simulink model "Lab07"  (R2024b)
settings: Solver=VariableStepAuto  StartTime=0.0  StopTime=10.0  RelTol=1e-3
values from neighbouring files (symbols this model uses):
  I = diag(Iv)    [initLab7.m]
  invI = inv(I)    [initLab7.m]
  w0 = [0; 0; 0]    [initLab7.m]
undefined symbols (not defined in the file or in its folder): env, IC, orb, sat, WMM2020
libraries: matrix_library x8, aerolibatmos2 x1, aerolibgravity2 x1
settings Model: Creator=elisa  LastModifiedBy=elisa
settings RTWCC: GPUComputeCapability=3.5

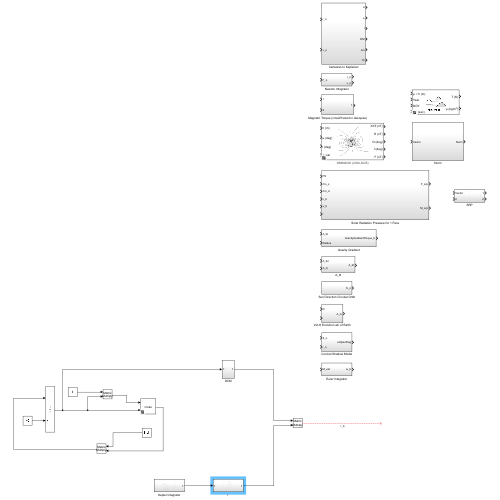
[thumbnail: Simulink's stored preview of the top-level diagram]
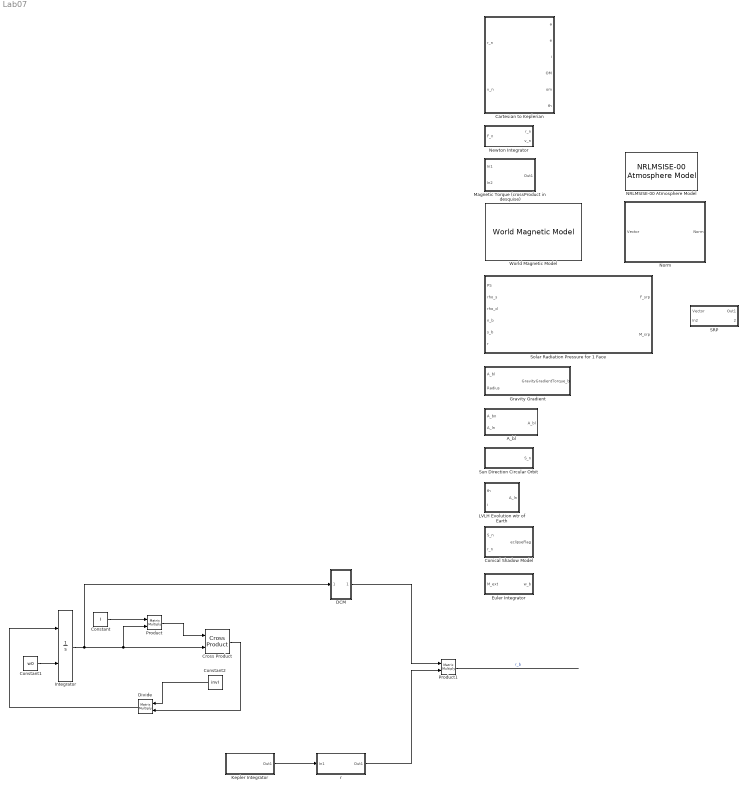
== system Lab07 ==
  A_bl : Subsystem
  Cartesian to Keplerian : Subsystem
  Conical Shadow Model : Subsystem
  Constant : Constant  Value=I
  Constant1 : Constant  Value=w0  VectorParams1D=off
  Constant2 : Constant  Value=invI
  Cross Product : matrix_library/Cross Product
  DCM : Subsystem
  Divide : Product  Inputs=**  Multiplication=Matrix(*)
  Euler Integrator : Subsystem
  Gravity Gradient : Subsystem
  Integrator : Integrator  InitialConditionSource=external
  Kepler Integrator : Subsystem
  LVLH Evolution wtr of Earth : Subsystem
  Magnetic Torque (crossProduct in desquise) : Subsystem
  NRLMSISE-00 Atmosphere Model : aerolibatmos2/NRLMSISE-00 Atmosphere Model  units=Metric (MKS)  lst_input=off  flux_ap_input=off  flags_input=Internal  flags=ones(1,23)  oxygen_in=off  action=Warning
  Newton Integrator : Subsystem
  Norm : Subsystem
  Product : Product  Multiplication=Matrix(*)
  Product1 : Product  Multiplication=Matrix(*)
  SRP : Subsystem
  Solar Radiation Pressure for 1 Face : Subsystem
  Sun Direction Circular Orbit : Subsystem
  World Magnetic Model : aerolibgravity2/World Magnetic Model  model=WMM2020 (2020-2025)  customFile='WMM2020.COF'  units=Metric (MKS)  time_in=on  month=January  day=1  year=2020  action=Error  h_out=on  dec_out=on  inc_out=on  ti_out=on
  r : Subsystem
  wires:
  Kepler Integrator/1(Out1) -> r/1(In1)
  Divide/1 -> Integrator/1
  Constant2/1 -> Divide/1
  Integrator/1 -> DCM/1(In1), Product/2, Cross Product/2
  Product/1 -> Cross Product/1
  Cross Product/1 -> Divide/2
  Constant1/1 -> Integrator/2
  Constant/1 -> Product/1
  DCM/1(Out1) -> Product1/1
  r/1(Out1) -> Product1/2
  Product1/1 -> ?  "r_b"

== system Lab07/A_bl ==
  A_bn : Inport
  A_ln : Inport  Port=2
  Matrix Multiply : Product  Multiplication=Matrix(*)
  Transpose : Math  Operator=transpose
  A_bl : Outport
  wires:
  Transpose/1 -> Matrix Multiply/2
  A_ln/1 -> Transpose/1
  Matrix Multiply/1 -> A_bl/1
  A_bn/1 -> Matrix Multiply/1

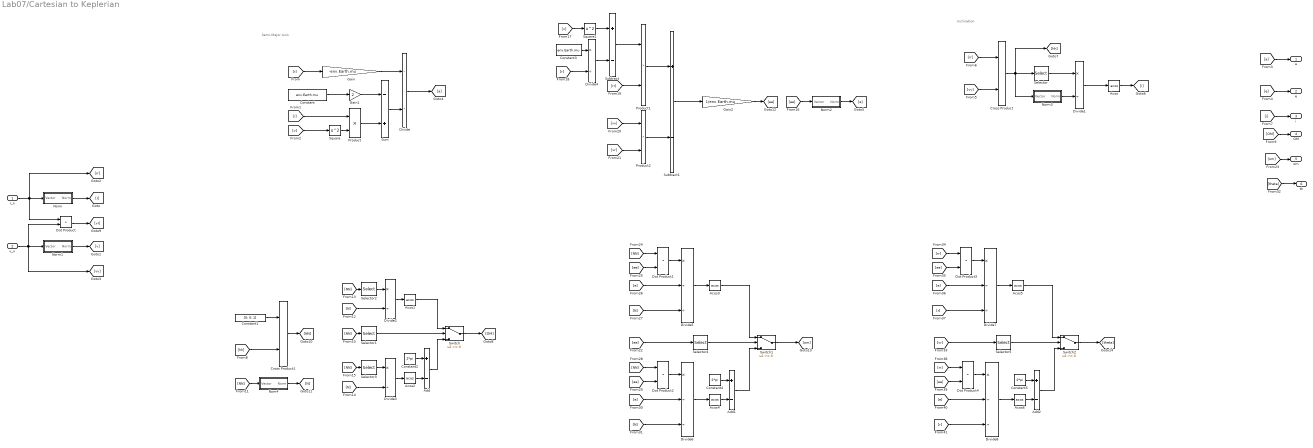
== system Lab07/Cartesian to Keplerian ==
  note: Semi-Major Axis
  note: Inclination
  r_n : Inport
  v_n : Inport  Port=2
  Acos{,1..6} (7 alike) : Trigonometry  Operator=acos
  Add : Sum  Inputs=+-
  Add1 : Sum  Inputs=+-
  Add2 : Sum  Inputs=+-
  Constant : Constant  Value=env.Earth.mu
  Constant1 : Constant  Value=[0; 0; 1]
  Constant2 : Constant  Value=2*pi
  Constant3 : Constant  Value=env.Earth.mu
  Constant4 : Constant  Value=2*pi
  Constant5 : Constant  Value=2*pi
  Cross Product : matrix_library/Cross Product
  Cross Product1 : matrix_library/Cross Product
  Divide{,1..4} (5 alike) : Product  Inputs=*/
  Divide{5..8} (4 alike) : Product  Inputs=*//
  Dot Product{,1..4} (5 alike) : DotProduct  OutDataTypeStr=Inherit: Inherit via internal rule
  Gain : Gain  Gain=-env.Earth.mu
  Gain1 : Gain  Gain=2
  Gain2 : Gain  Gain=1/env.Earth.mu
  Nom4 : Subsystem
  Norm : Subsystem
  Norm1 : Subsystem
  Norm2 : Subsystem
  Norm3 : Subsystem
  Product : Product
  Product1 : Product
  Product2 : Product
  Selector : Selector  InputPortWidth=3  IndexOptions=Index vector (dialog)  Indices=[3]  OutputSizes=1
  Selector1 : Selector  InputPortWidth=3  IndexOptions=Index vector (dialog)  Indices=[2]  OutputSizes=1
  Selector2 : Selector  InputPortWidth=3  IndexOptions=Index vector (dialog)  Indices=[1]  OutputSizes=1
  Selector3 : Selector  InputPortWidth=3  IndexOptions=Index vector (dialog)  Indices=[1]  OutputSizes=1
  Selector4 : Selector  InputPortWidth=3  IndexOptions=Index vector (dialog)  Indices=3  OutputSizes=1
  Selector5 : Selector  InputPortWidth=3  IndexOptions=Index vector (dialog)  Indices=3  OutputSizes=1
  Square : Math  Operator=square
  Square1 : Math  Operator=square
  Subtract : Sum  Inputs=+-
  Subtract1 : Sum  Inputs=+-
  Sum : Sum  Inputs=-+
  Switch : Switch  SaturateOnIntegerOverflow=off  InputSameDT=off
  Switch1 : Switch  SaturateOnIntegerOverflow=off  InputSameDT=off
  Switch2 : Switch  SaturateOnIntegerOverflow=off  InputSameDT=off
  a : Outport
  e : Outport  Port=2
  i : Outport  Port=3
  OM : Outport  Port=4
  om : Outport  Port=5
  th : Outport  Port=6
  wires:
  r_n/1 -> Dot Product/1, [rr], Norm/1(Vector)
  v_n/1 -> Dot Product/2, [vv], Norm1/1(Vector)
  Norm/1(Norm) -> [r]
  Norm1/1(Norm) -> [v]
  Gain/1 -> Divide/1
  [r] -> Gain/1
  Sum/1 -> Divide/2
  Constant/1 -> Gain1/1
  Gain1/1 -> Sum/1
  Product/1 -> Sum/2
  [r] -> Product/1
  Square/1 -> Product/2
  [v] -> Square/1
  Divide/1 -> [a]
  [a] -> a/1
  Norm2/1(Norm) -> [e]
  [e] -> e/1
  [vv] -> Cross Product/2
  [rr] -> Cross Product/1
  Cross Product/1 -> [hh], Norm3/1(Vector), Selector/1
  Selector/1 -> Divide1/1
  Norm3/1(Norm) -> Divide1/2
  Divide1/1 -> Acos/1
  Acos/1 -> [i]
  [i] -> i/1
  [hh] -> Cross Product1/2
  Constant1/1 -> Cross Product1/1
  Selector1/1 -> Switch/2
  [OM] -> OM/1
  Switch/1 -> [OM]
  Dot Product/1 -> [vr]
  Cross Product1/1 -> [NN]
  [NN] -> Selector1/1
  [NN] -> Nom4/1(Vector)
  Nom4/1(Norm) -> [N]
  [NN] -> Selector2/1
  [N] -> Divide2/2
  Selector2/1 -> Divide2/1
  Acos1/1 -> Switch/1
  Selector3/1 -> Divide3/1
  [NN] -> Selector3/1
  [N] -> Divide3/2
  Divide3/1 -> Acos2/1
  Divide2/1 -> Acos1/1
  Acos2/1 -> Add/2
  Constant2/1 -> Add/1
  Add/1 -> Switch/3
  [ee] -> Norm2/1(Vector)
  Gain2/1 -> [ee]
  [v] -> Square1/1
  Constant3/1 -> Divide4/1
  [r] -> Divide4/2
  Divide4/1 -> Subtract/2
  Square1/1 -> Subtract/1
  Subtract/1 -> Product1/1
  [rr] -> Product1/2
  Product1/1 -> Subtract1/1
  Product2/1 -> Subtract1/2
  [vv] -> Product2/1
  [vr] -> Product2/2
  Subtract1/1 -> Gain2/1
  Selector4/1 -> Switch1/2
  [ee] -> Selector4/1
  Switch1/1 -> [om]
  [om] -> om/1
  [NN] -> Dot Product1/1
  [ee] -> Dot Product1/2
  Dot Product1/1 -> Divide5/1
  [e] -> Divide5/2
  [N] -> Divide5/3
  Divide5/1 -> Acos3/1
  Acos3/1 -> Switch1/1
  [ee] -> Dot Product2/2
  Divide6/1 -> Acos4/1
  Dot Product2/1 -> Divide6/1
  [NN] -> Dot Product2/1
  [N] -> Divide6/3
  [e] -> Divide6/2
  Constant4/1 -> Add1/1
  Acos4/1 -> Add1/2
  Add1/1 -> Switch1/3
  [vr] -> Selector5/1
  Switch2/1 -> [theta]
  Selector5/1 -> Switch2/2
  [theta] -> th/1
  [ee] -> Dot Product3/2
  Divide7/1 -> Acos5/1
  Dot Product3/1 -> Divide7/1
  [rr] -> Dot Product3/1
  [r] -> Divide7/3
  Acos5/1 -> Switch2/1
  [e] -> Divide7/2
  Add2/1 -> Switch2/3
  [rr] -> Dot Product4/1
  [r] -> Divide8/3
  Dot Product4/1 -> Divide8/1
  [e] -> Divide8/2
  Acos6/1 -> Add2/2
  Constant5/1 -> Add2/1
  Divide8/1 -> Acos6/1
  [ee] -> Dot Product4/2

== system Lab07/Conical Shadow Model ==
  note: Output Interface
  note: Input Interface
  note: Model is cylindrical shadow, formula was taken by Crassidis
  S_n : Inport
  r_n : Inport  Port=2
  Dot Product : DotProduct  OutDataTypeStr=Inherit: Inherit via internal rule
  Earth's Radius : Constant  Value=env.Earth.R
  Eclipse (1) : Subsystem  TreatAsAtomicUnit=on
  Gain : Gain  Gain=-1
  If : If  NumInputs=2  IfExpression=u1 < u2
  Merge : Merge
  Norm : Subsystem
  NotEclipse (0) : Subsystem  TreatAsAtomicUnit=on
  Sqrt : Sqrt
  Square : Math  Operator=square
  Square1 : Math  Operator=square
  Subtract : Sum  Inputs=+-
  eclipseFlag : Outport
  wires:
  r_n/1 -> Dot Product/2, Norm/1(Vector)  "r_n"
  S_n/1 -> Dot Product/1  "S_n"
  Norm/1(Norm) -> Square1/1  "norm_r"
  If/1 -> Eclipse (1)/Action
  If/2 -> NotEclipse (0)/Action
  Merge/1 -> eclipseFlag/1
  Eclipse (1)/1(One) -> Merge/1
  NotEclipse (0)/1(Zero) -> Merge/2
  Dot Product/1 -> If/1
  Gain/1 -> If/2
  Sqrt/1 -> Gain/1
  Subtract/1 -> Sqrt/1
  Square/1 -> Subtract/2
  Square1/1 -> Subtract/1
  Earth's Radius/1 -> Square/1  "earth_R"

== system Lab07/DCM ==
  In1 : Inport
  A312 : Subsystem
  Constant3 : Constant  Value=IC.angles
  Gain : Gain  Gain=-1
  Integrator1 : Integrator  InitialConditionSource=external
  Product1 : Product  Multiplication=Matrix(*)
  Subsystem : Subsystem
  Subsystem1 : Subsystem
  Subsystem2 : Subsystem
  w^ : Subsystem
  Out1 : Outport
  wires:
  w^/1(Out1) -> Gain/1
  Gain/1 -> Product1/1
  In1/1 -> w^/1(In1)
  Product1/1 -> Integrator1/1
  Constant3/1 -> A312/1(In1)
  Integrator1/1 -> Subsystem/1(In1)
  Subsystem/1(Out1) -> Subsystem1/1(In1)
  A312/1(Out1) -> Integrator1/2
  Subsystem1/1(Out1) -> Subsystem2/1(In1)
  Subsystem2/1(Out1) -> Product1/2, Out1/1

== system Lab07/Euler Integrator ==
  M_ext : Inport
  Constant : Constant  Value=I
  Constant1 : Constant  Value=w0  VectorParams1D=off
  Constant2 : Constant  Value=invI
  Cross Product : matrix_library/Cross Product
  Divide : Product  Inputs=**  Multiplication=Matrix(*)
  Integrator : Integrator  InitialConditionSource=external
  Product : Product  Multiplication=Matrix(*)
  Sum : Sum  Inputs=|++
  w_b : Outport
  wires:
  Product/1 -> Cross Product/1
  Divide/1 -> Integrator/1
  Constant/1 -> Product/1
  Constant2/1 -> Divide/1
  Integrator/1 -> Product/2, Cross Product/2, w_b/1
  Constant1/1 -> Integrator/2
  Cross Product/1 -> Sum/1
  Sum/1 -> Divide/2
  M_ext/1 -> Sum/2

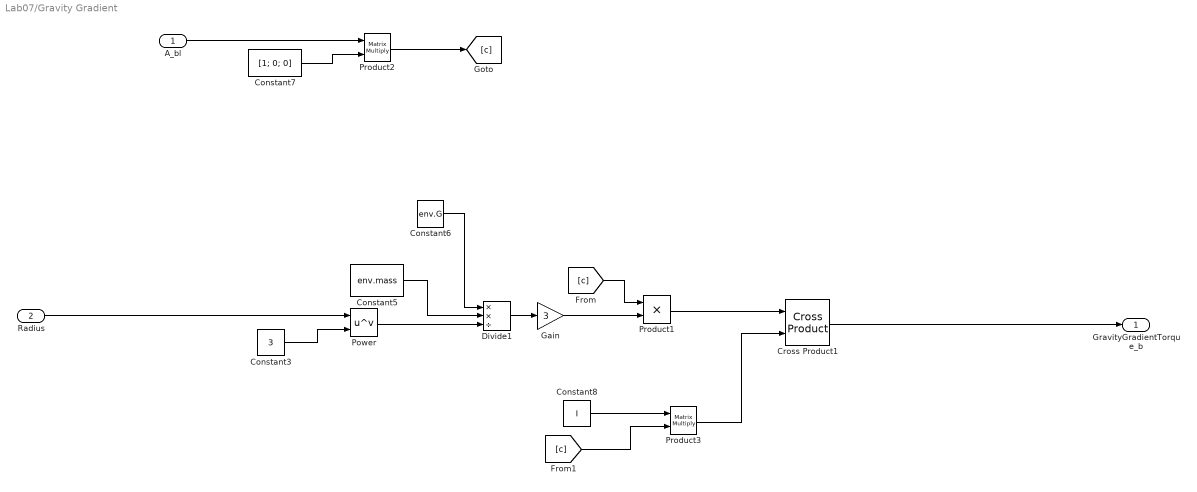
== system Lab07/Gravity Gradient ==
  A_bl : Inport
  Radius : Inport  Port=2
  Constant3 : Constant  Value=3
  Constant5 : Constant  Value=env.mass
  Constant6 : Constant  Value=env.G
  Constant7 : Constant  Value=[1; 0; 0]  VectorParams1D=off
  Constant8 : Constant  Value=I
  Cross Product1 : matrix_library/Cross Product
  Divide1 : Product  Inputs=**/
  Gain : Gain  Gain=3
  Power : Math  Operator=pow
  Product1 : Product
  Product2 : Product  Multiplication=Matrix(*)
  Product3 : Product  Multiplication=Matrix(*)
  GravityGradientTorque_b : Outport
  wires:
  Divide1/1 -> Gain/1
  Power/1 -> Divide1/3
  Constant3/1 -> Power/2
  Constant7/1 -> Product2/2
  Radius/1 -> Power/1
  Constant5/1 -> Divide1/2
  Constant6/1 -> Divide1/1
  [c] -> Product3/2
  [c] -> Product1/1
  Product1/1 -> Cross Product1/1
  Cross Product1/1 -> GravityGradientTorque_b/1
  Constant8/1 -> Product3/1
  Product2/1 -> [c]
  Product3/1 -> Cross Product1/2
  A_bl/1 -> Product2/1
  Gain/1 -> Product1/2

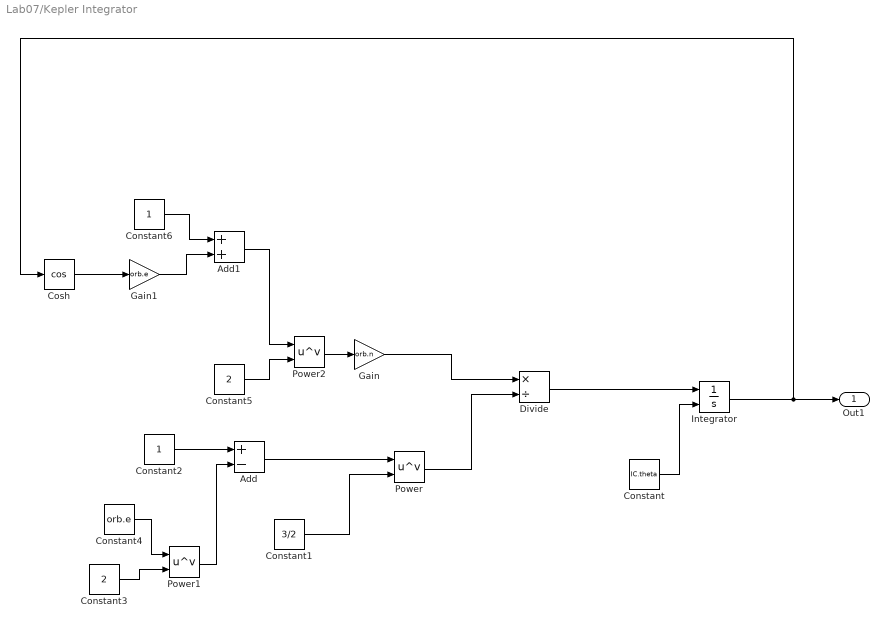
== system Lab07/Kepler Integrator ==
  Add : Sum  Inputs=+-
  Add1 : Sum
  Constant : Constant  Value=IC.theta
  Constant1 : Constant  Value=3/2
  Constant2 : Constant
  Constant3 : Constant  Value=2
  Constant4 : Constant  Value=orb.e
  Constant5 : Constant  Value=2
  Constant6 : Constant
  Cosh : Trigonometry  Operator=cos
  Divide : Product  Inputs=*/
  Gain : Gain  Gain=orb.n
  Gain1 : Gain  Gain=orb.e
  Integrator : Integrator  InitialConditionSource=external  WrapState=on  WrappedStateUpperValue=2*pi  WrappedStateLowerValue=0
  Power : Math  Operator=pow
  Power1 : Math  Operator=pow
  Power2 : Math  Operator=pow
  Out1 : Outport
  wires:
  Constant/1 -> Integrator/2
  Integrator/1 -> Cosh/1, Out1/1
  Divide/1 -> Integrator/1
  Power/1 -> Divide/2
  Constant1/1 -> Power/2
  Constant2/1 -> Add/1
  Add/1 -> Power/1
  Power1/1 -> Add/2
  Constant3/1 -> Power1/2
  Constant4/1 -> Power1/1
  Gain/1 -> Divide/1
  Power2/1 -> Gain/1
  Constant5/1 -> Power2/2
  Add1/1 -> Power2/1
  Constant6/1 -> Add1/1
  Gain1/1 -> Add1/2
  Cosh/1 -> Gain1/1

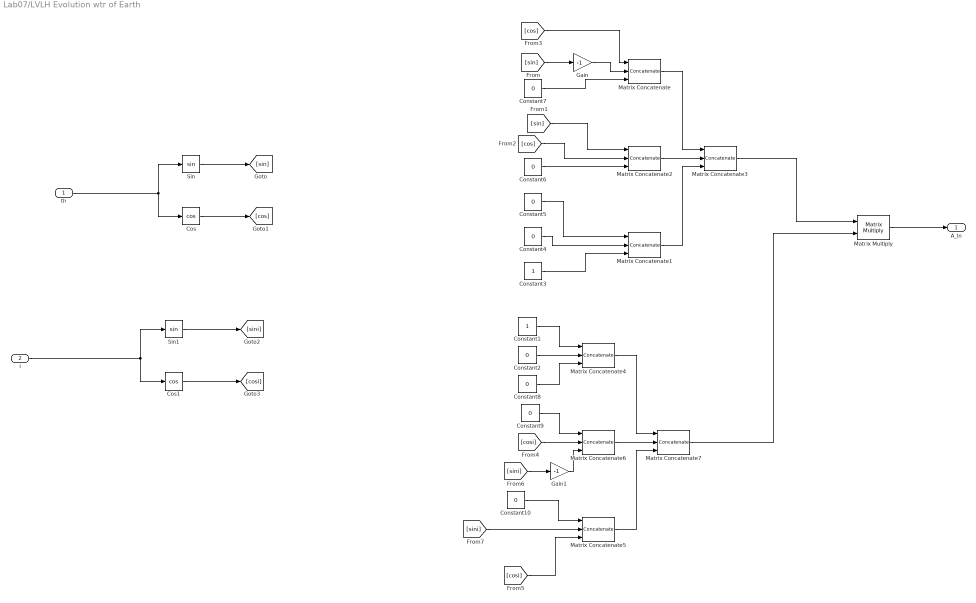
== system Lab07/LVLH Evolution wtr of Earth ==
  th : Inport
  i : Inport  Port=2
  Constant1 : Constant
  Constant{2,4..10} (8 alike) : Constant  Value=0
  Constant3 : Constant
  Cos : Trigonometry  Operator=cos
  Cos1 : Trigonometry  Operator=cos
  Gain : Gain  Gain=-1
  Gain1 : Gain  Gain=-1
  Matrix Concatenate{,1..2,4..6} (6 alike) : Concatenate  NumInputs=3  Mode=Multidimensional array
  Matrix Concatenate3 : Concatenate  NumInputs=3  Mode=Multidimensional array  ConcatenateDimension=2
  Matrix Concatenate7 : Concatenate  NumInputs=3  Mode=Multidimensional array  ConcatenateDimension=2
  Matrix Multiply : Product  Multiplication=Matrix(*)
  Sin : Trigonometry
  Sin1 : Trigonometry
  A_ln : Outport
  wires:
  Cos/1 -> [cos]
  Matrix Concatenate1/1 -> Matrix Concatenate3/3
  th/1 -> Cos/1, Sin/1
  Matrix Concatenate/1 -> Matrix Concatenate3/1
  Constant5/1 -> Matrix Concatenate1/1
  Constant3/1 -> Matrix Concatenate1/3
  [cos] -> Matrix Concatenate/1
  Sin/1 -> [sin]
  Constant6/1 -> Matrix Concatenate2/3
  Constant7/1 -> Matrix Concatenate/3
  Constant4/1 -> Matrix Concatenate1/2
  Matrix Concatenate2/1 -> Matrix Concatenate3/2
  [cos] -> Matrix Concatenate2/2
  [sin] -> Matrix Concatenate2/1
  Gain/1 -> Matrix Concatenate/2
  [sin] -> Gain/1
  Cos1/1 -> [cosi]
  Sin1/1 -> [sini]
  i/1 -> Cos1/1, Sin1/1
  Matrix Multiply/1 -> A_ln/1
  Matrix Concatenate3/1 -> Matrix Multiply/1
  Matrix Concatenate7/1 -> Matrix Multiply/2
  Matrix Concatenate6/1 -> Matrix Concatenate7/2
  Matrix Concatenate5/1 -> Matrix Concatenate7/3
  Matrix Concatenate4/1 -> Matrix Concatenate7/1
  Constant1/1 -> Matrix Concatenate4/1
  Constant2/1 -> Matrix Concatenate4/2
  Constant8/1 -> Matrix Concatenate4/3
  Constant9/1 -> Matrix Concatenate6/1
  Constant10/1 -> Matrix Concatenate5/1
  [cosi] -> Matrix Concatenate5/3
  [cosi] -> Matrix Concatenate6/2
  [sini] -> Matrix Concatenate5/2
  [sini] -> Gain1/1
  Gain1/1 -> Matrix Concatenate6/3

== system Lab07/Magnetic Torque (crossProduct in desquise) ==
  In1 : Inport
  In2 : Inport  Port=2
  Cross Product : matrix_library/Cross Product
  Out1 : Outport
  wires:
  Cross Product/1 -> Out1/1
  In1/1 -> Cross Product/1
  In2/1 -> Cross Product/2

== system Lab07/Newton Integrator ==
  F_n : Inport
  Constant : Constant  Value=IC.velocity
  Constant1 : Constant  Value=IC.position
  Constant2 : Constant  Value=sat.mass
  Divide : Product  Inputs=*/
  Integrator : Integrator  InitialConditionSource=external
  Integrator1 : Integrator  InitialConditionSource=external
  r_n : Outport
  v_n : Outport  Port=2
  wires:
  Integrator/1 -> r_n/1, Integrator1/1
  Integrator1/1 -> v_n/1
  Constant/1 -> Integrator/2
  Constant1/1 -> Integrator1/2
  F_n/1 -> Divide/1
  Divide/1 -> Integrator/1
  Constant2/1 -> Divide/2

== system Lab07/Norm ==
  Vector : Inport
  Add : Sum  Inputs=+++
  Demux : Demux  Outputs=3
  Sqrt : Sqrt
  Square : Math  Operator=square
  Square1 : Math  Operator=square
  Square2 : Math  Operator=square
  Norm : Outport
  wires:
  Square/1 -> Add/1
  Add/1 -> Sqrt/1
  Demux/3 -> Square1/1
  Square2/1 -> Add/2
  Square1/1 -> Add/3
  Demux/1 -> Square/1
  Demux/2 -> Square2/1
  Vector/1 -> Demux/1
  Sqrt/1 -> Norm/1

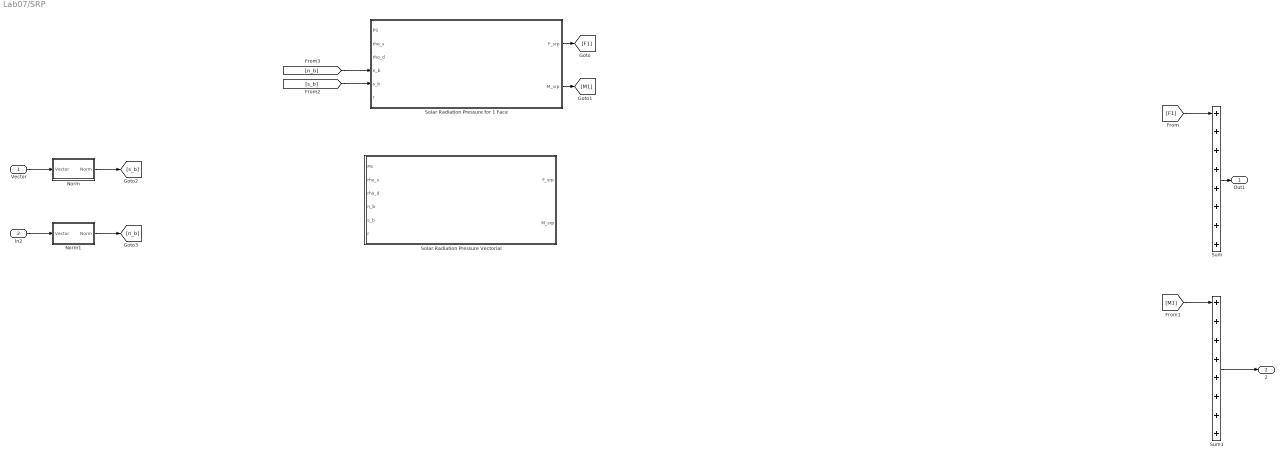
== system Lab07/SRP ==
  Vector : Inport
  In2 : Inport  Port=2
  Norm : Subsystem
  Norm1 : Subsystem
  Solar Radiation Pressure Vectorial : Subsystem
  Solar Radiation Pressure for 1 Face : Subsystem
  Sum : Sum  Inputs=++++++++
  Sum1 : Sum  Inputs=++++++++
  Out1 : Outport
  2 : Outport  Port=2
  wires:
  Sum/1 -> Out1/1
  Sum1/1 -> 2/1
  Solar Radiation Pressure for 1 Face/1(F_srp) -> [F1]
  [F1] -> Sum/1
  Solar Radiation Pressure for 1 Face/2(M_srp) -> [M1]
  [M1] -> Sum1/1
  Vector/1 -> Norm/1(Vector)
  In2/1 -> Norm1/1(Vector)
  Norm/1(Norm) -> [s_b]
  Norm1/1(Norm) -> [n_b]
  [s_b] -> Solar Radiation Pressure for 1 Face/5(s_b)
  [n_b] -> Solar Radiation Pressure for 1 Face/4(n_b)

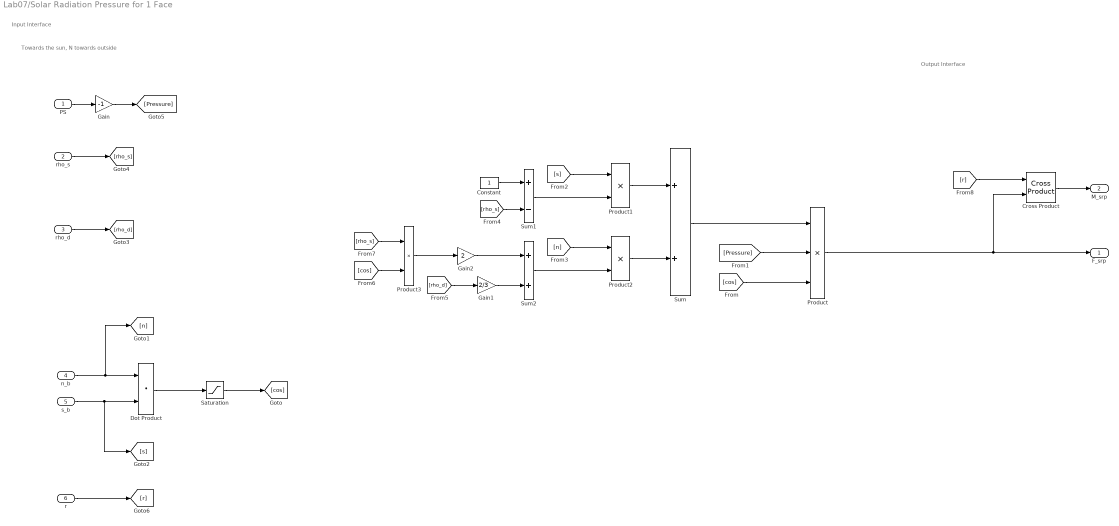
== system Lab07/Solar Radiation Pressure for 1 Face ==
  note: Towards the sun, N towards outside
  note: Output Interface
  note: Input Interface
  PS : Inport
  rho_s : Inport  Port=2
  rho_d : Inport  Port=3
  n_b : Inport  Port=4
  s_b : Inport  Port=5
  r : Inport  Port=6
  Constant : Constant
  Cross Product : matrix_library/Cross Product
  Dot Product : DotProduct  OutDataTypeStr=Inherit: Inherit via internal rule
  Gain : Gain  Gain=-1
  Gain1 : Gain  Gain=2/3
  Gain2 : Gain  Gain=2
  Product : Product  Inputs=3
  Product1 : Product
  Product2 : Product
  Product3 : Product
  Saturation : Saturate  UpperLimit=1  LowerLimit=0
  Sum : Sum
  Sum1 : Sum  Inputs=+-
  Sum2 : Sum
  F_srp : Outport
  M_srp : Outport  Port=2
  wires:
  s_b/1 -> [s], Dot Product/2
  n_b/1 -> [n], Dot Product/1
  Dot Product/1 -> Saturation/1
  Saturation/1 -> [cos]
  PS/1 -> Gain/1
  Product/1 -> Cross Product/2, F_srp/1
  rho_d/1 -> [rho_d]
  rho_s/1 -> [rho_s]
  [cos] -> Product/3
  Gain/1 -> [Pressure]
  [Pressure] -> Product/2
  Sum/1 -> Product/1
  [s] -> Product1/1
  Product1/1 -> Sum/1
  Product2/1 -> Sum/2
  [n] -> Product2/1
  Sum1/1 -> Product1/2
  Sum2/1 -> Product2/2
  Constant/1 -> Sum1/1
  [rho_s] -> Sum1/2
  Gain1/1 -> Sum2/2
  [rho_d] -> Gain1/1
  Gain2/1 -> Sum2/1
  Product3/1 -> Gain2/1
  [cos] -> Product3/2
  [rho_s] -> Product3/1
  r/1 -> [r]
  [r] -> Cross Product/1
  Cross Product/1 -> M_srp/1

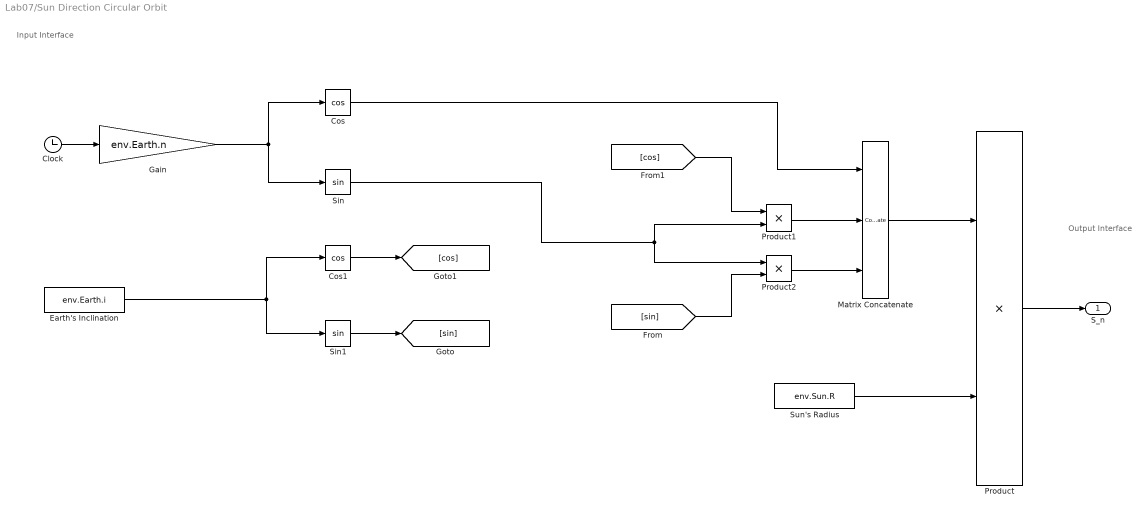
== system Lab07/Sun Direction Circular Orbit ==
  note: Input Interface
  note: Output Interface
  Clock : Clock
  Cos : Trigonometry  Operator=cos
  Cos1 : Trigonometry  Operator=cos
  Earth's Inclination : Constant  Value=env.Earth.i
  Gain : Gain  Gain=env.Earth.n
  Matrix Concatenate : Concatenate  NumInputs=3  Mode=Multidimensional array
  Product : Product
  Product1 : Product
  Product2 : Product
  Sin : Trigonometry
  Sin1 : Trigonometry
  Sun's Radius : Constant  Value=env.Sun.R
  S_n : Outport
  wires:
  Clock/1 -> Gain/1
  Gain/1 -> Sin/1, Cos/1
  Product/1 -> S_n/1
  Sun's Radius/1 -> Product/2
  Matrix Concatenate/1 -> Product/1
  Earth's Inclination/1 -> Sin1/1, Cos1/1
  Cos1/1 -> [cos]
  Sin1/1 -> [sin]
  Cos/1 -> Matrix Concatenate/1
  Product1/1 -> Matrix Concatenate/2
  Product2/1 -> Matrix Concatenate/3
  [sin] -> Product2/2
  [cos] -> Product1/1
  Sin/1 -> Product1/2, Product2/1

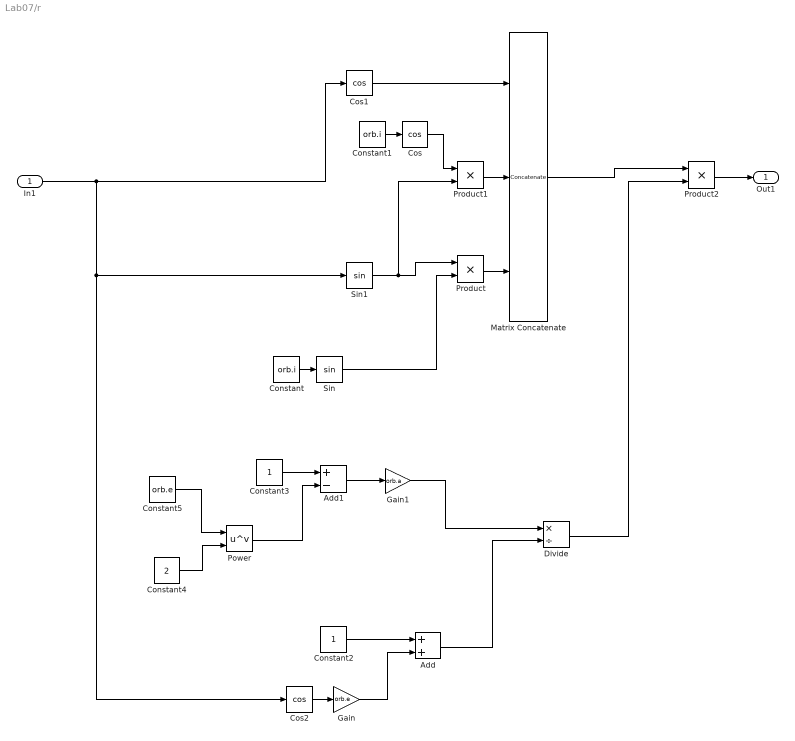
== system Lab07/r ==
  In1 : Inport
  Add : Sum
  Add1 : Sum  Inputs=+-
  Constant : Constant  Value=orb.i
  Constant1 : Constant  Value=orb.i
  Constant2 : Constant
  Constant3 : Constant
  Constant4 : Constant  Value=2
  Constant5 : Constant  Value=orb.e
  Cos : Trigonometry  Operator=cos
  Cos1 : Trigonometry  Operator=cos
  Cos2 : Trigonometry  Operator=cos
  Divide : Product  Inputs=*/
  Gain : Gain  Gain=orb.e
  Gain1 : Gain  Gain=orb.a
  Matrix Concatenate : Concatenate  NumInputs=3  Mode=Multidimensional array
  Power : Math  Operator=pow
  Product : Product
  Product1 : Product
  Product2 : Product
  Sin : Trigonometry
  Sin1 : Trigonometry
  Out1 : Outport
  wires:
  Constant/1 -> Sin/1
  Cos1/1 -> Matrix Concatenate/1
  In1/1 -> Sin1/1, Cos2/1, Cos1/1
  Product1/1 -> Matrix Concatenate/2
  Product/1 -> Matrix Concatenate/3
  Sin1/1 -> Product1/2, Product/1
  Sin/1 -> Product/2
  Constant1/1 -> Cos/1
  Cos/1 -> Product1/1
  Product2/1 -> Out1/1
  Matrix Concatenate/1 -> Product2/1
  Divide/1 -> Product2/2
  Constant2/1 -> Add/1
  Add/1 -> Divide/2
  Cos2/1 -> Gain/1
  Gain/1 -> Add/2
  Constant3/1 -> Add1/1
  Power/1 -> Add1/2
  Constant4/1 -> Power/2
  Constant5/1 -> Power/1
  Add1/1 -> Gain1/1
  Gain1/1 -> Divide/1

== system Lab07/Cartesian to Keplerian/Nom4 ==
  Vector : Inport
  Add : Sum  Inputs=+++
  Demux : Demux  Outputs=3
  Sqrt : Sqrt
  Square : Math  Operator=square
  Square1 : Math  Operator=square
  Square2 : Math  Operator=square
  Norm : Outport
  wires:
  Square/1 -> Add/1
  Add/1 -> Sqrt/1
  Demux/3 -> Square1/1
  Square2/1 -> Add/2
  Square1/1 -> Add/3
  Demux/1 -> Square/1
  Demux/2 -> Square2/1
  Vector/1 -> Demux/1
  Sqrt/1 -> Norm/1

== system Lab07/Cartesian to Keplerian/Norm ==
  Vector : Inport
  Add : Sum  Inputs=+++
  Demux : Demux  Outputs=3
  Sqrt : Sqrt
  Square : Math  Operator=square
  Square1 : Math  Operator=square
  Square2 : Math  Operator=square
  Norm : Outport
  wires:
  Square/1 -> Add/1
  Add/1 -> Sqrt/1
  Demux/3 -> Square1/1
  Square2/1 -> Add/2
  Square1/1 -> Add/3
  Demux/1 -> Square/1
  Demux/2 -> Square2/1
  Vector/1 -> Demux/1
  Sqrt/1 -> Norm/1

== system Lab07/Cartesian to Keplerian/Norm1 ==
  Vector : Inport
  Add : Sum  Inputs=+++
  Demux : Demux  Outputs=3
  Sqrt : Sqrt
  Square : Math  Operator=square
  Square1 : Math  Operator=square
  Square2 : Math  Operator=square
  Norm : Outport
  wires:
  Square/1 -> Add/1
  Add/1 -> Sqrt/1
  Demux/3 -> Square1/1
  Square2/1 -> Add/2
  Square1/1 -> Add/3
  Demux/1 -> Square/1
  Demux/2 -> Square2/1
  Vector/1 -> Demux/1
  Sqrt/1 -> Norm/1

== system Lab07/Cartesian to Keplerian/Norm2 ==
  Vector : Inport
  Add : Sum  Inputs=+++
  Demux : Demux  Outputs=3
  Sqrt : Sqrt
  Square : Math  Operator=square
  Square1 : Math  Operator=square
  Square2 : Math  Operator=square
  Norm : Outport
  wires:
  Square/1 -> Add/1
  Add/1 -> Sqrt/1
  Demux/3 -> Square1/1
  Square2/1 -> Add/2
  Square1/1 -> Add/3
  Demux/1 -> Square/1
  Demux/2 -> Square2/1
  Vector/1 -> Demux/1
  Sqrt/1 -> Norm/1

== system Lab07/Cartesian to Keplerian/Norm3 ==
  Vector : Inport
  Add : Sum  Inputs=+++
  Demux : Demux  Outputs=3
  Sqrt : Sqrt
  Square : Math  Operator=square
  Square1 : Math  Operator=square
  Square2 : Math  Operator=square
  Norm : Outport
  wires:
  Square/1 -> Add/1
  Add/1 -> Sqrt/1
  Demux/3 -> Square1/1
  Square2/1 -> Add/2
  Square1/1 -> Add/3
  Demux/1 -> Square/1
  Demux/2 -> Square2/1
  Vector/1 -> Demux/1
  Sqrt/1 -> Norm/1

== system Lab07/Conical Shadow Model/Eclipse (1) ==
  Action Port : ActionPort  ActionPortLabel=if(u1 > 0)
  Constant : Constant
  One : Outport
  wires:
  Constant/1 -> One/1

== system Lab07/Conical Shadow Model/Norm ==
  Vector : Inport
  Add : Sum  Inputs=+++
  Demux : Demux  Outputs=3
  Sqrt : Sqrt
  Square : Math  Operator=square
  Square1 : Math  Operator=square
  Square2 : Math  Operator=square
  Norm : Outport
  wires:
  Square/1 -> Add/1
  Add/1 -> Sqrt/1
  Demux/3 -> Square1/1
  Square2/1 -> Add/2
  Square1/1 -> Add/3
  Demux/1 -> Square/1
  Demux/2 -> Square2/1
  Vector/1 -> Demux/1
  Sqrt/1 -> Norm/1

== system Lab07/Conical Shadow Model/NotEclipse (0) ==
  Action Port : ActionPort  ActionPortLabel=else
  Constant : Constant  Value=0
  Zero : Outport
  wires:
  Constant/1 -> Zero/1

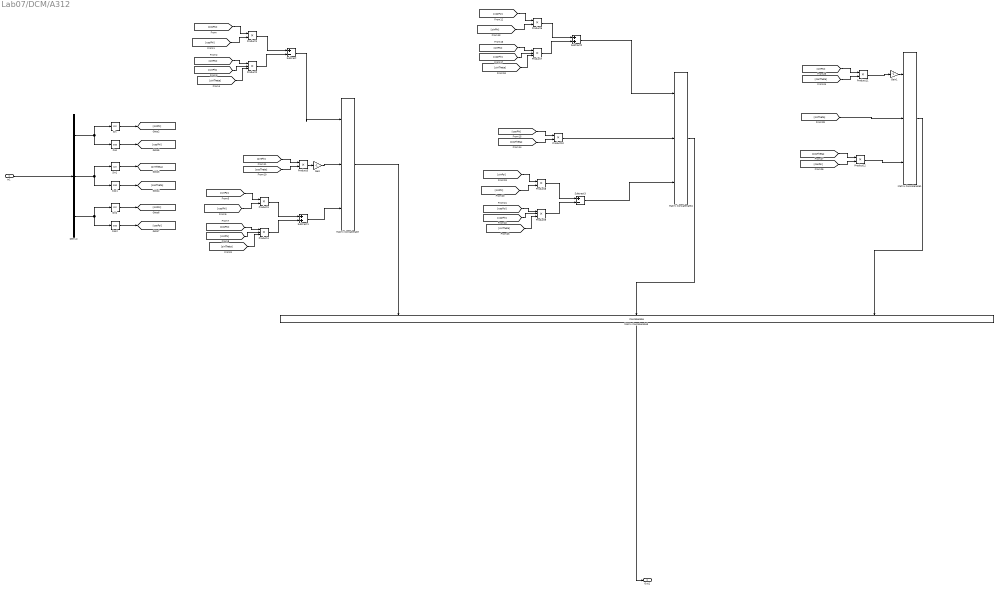
== system Lab07/DCM/A312 ==
  In1 : Inport
  Cos : Trigonometry  Operator=cos
  Cos1 : Trigonometry  Operator=cos
  Cos2 : Trigonometry  Operator=cos
  Demux : Demux  Outputs=3
  Gain : Gain  Gain=-1
  Gain1 : Gain  Gain=-1
  Matrix Concatenate : Concatenate  NumInputs=3  Mode=Multidimensional array
  Matrix Concatenate1 : Concatenate  NumInputs=3  Mode=Multidimensional array
  Matrix Concatenate3 : Concatenate  NumInputs=3  Mode=Multidimensional array  ConcatenateDimension=2
  Matrix Concatenate4 : Concatenate  NumInputs=3  Mode=Multidimensional array
  Product{1,3,5..6,8,10..12} (8 alike) : Product
  Product{2,4,7,9} (4 alike) : Product  Inputs=3
  Sin : Trigonometry
  Sin1 : Trigonometry
  Sin2 : Trigonometry
  Subtract : Sum  Inputs=+-
  Subtract1 : Sum
  Subtract2 : Sum
  Subtract3 : Sum  Inputs=+-
  Out1 : Outport
  wires:
  In1/1 -> Demux/1
  [sinTheta] -> Product2/3
  Product7/1 -> Subtract2/2
  [cosTheta] -> Product11/2
  [sinPhi] -> Product8/2
  Sin/1 -> [sinPhi]
  [sinPhi] -> Product2/2
  [cosTheta] -> Product10/2
  [cosPsi] -> Product6/1
  Demux/3 -> Sin2/1, Cos2/1
  Product9/1 -> Subtract3/2
  [sinTheta] -> Matrix Concatenate1/2
  Matrix Concatenate1/1 -> Matrix Concatenate3/3
  [sinPsi] -> Product11/1
  Product2/1 -> Subtract/2
  Subtract2/1 -> Matrix Concatenate4/1
  Matrix Concatenate4/1 -> Matrix Concatenate3/2
  [cosTheta] -> Product12/1
  Cos2/1 -> [cosPsi]
  [sinPsi] -> Product2/1
  [sinPsi] -> Product8/1
  Sin2/1 -> [sinPsi]
  [sinTheta] -> Product7/3
  Subtract/1 -> Matrix Concatenate/1
  [cosPhi] -> Product10/1
  Demux/2 -> Sin1/1, Cos1/1
  [sinTheta] -> Product9/3
  Product8/1 -> Subtract3/1
  [cosPhi] -> Product9/2
  [cosPsi] -> Product9/1
  Product11/1 -> Gain1/1
  Product1/1 -> Subtract/1
  [cosPhi] -> Product1/2
  [cosPsi] -> Product12/2
  [cosPhi] -> Product7/2
  [sinPhi] -> Product6/2
  Product6/1 -> Subtract2/1
  Demux/1 -> Sin/1, Cos/1
  [cosPsi] -> Product1/1
  [sinPsi] -> Product7/1
  Cos1/1 -> [cosTheta]
  Sin1/1 -> [sinTheta]
  Product12/1 -> Matrix Concatenate1/3
  Matrix Concatenate/1 -> Matrix Concatenate3/1
  Cos/1 -> [cosPhi]
  Matrix Concatenate3/1 -> Out1/1
  Gain1/1 -> Matrix Concatenate1/1
  Product10/1 -> Matrix Concatenate4/2
  Subtract3/1 -> Matrix Concatenate4/3
  [cosPsi] -> Product4/1
  Product4/1 -> Subtract1/2
  [cosPhi] -> Product3/2
  Product3/1 -> Subtract1/1
  [sinPsi] -> Product3/1
  [sinPhi] -> Product4/2
  [sinTheta] -> Product4/3
  [sinPhi] -> Product5/1
  [cosTheta] -> Product5/2
  Product5/1 -> Gain/1
  Subtract1/1 -> Matrix Concatenate/3
  Gain/1 -> Matrix Concatenate/2

== system Lab07/DCM/Subsystem ==
  In1 : Inport
  Gain1 : Gain  Gain=3/2
  Gain2 : Gain  Gain=1/2
  Product : Product  Inputs=3  Multiplication=Matrix(*)
  Subtract : Sum  Inputs=+-
  Transpose : Math  Operator=transpose
  Out1 : Outport
  wires:
  In1/1 -> Product/3, Product/1, Gain1/1, Transpose/1
  Gain2/1 -> Subtract/2
  Gain1/1 -> Subtract/1
  Product/1 -> Gain2/1
  Transpose/1 -> Product/2
  Subtract/1 -> Out1/1

== system Lab07/DCM/Subsystem1 ==
  In1 : Inport
  Gain1 : Gain  Gain=3/2
  Gain2 : Gain  Gain=1/2
  Product : Product  Inputs=3  Multiplication=Matrix(*)
  Subtract : Sum  Inputs=+-
  Transpose : Math  Operator=transpose
  Out1 : Outport
  wires:
  In1/1 -> Product/3, Product/1, Gain1/1, Transpose/1
  Gain2/1 -> Subtract/2
  Gain1/1 -> Subtract/1
  Product/1 -> Gain2/1
  Transpose/1 -> Product/2
  Subtract/1 -> Out1/1

== system Lab07/DCM/Subsystem2 ==
  In1 : Inport
  Gain1 : Gain  Gain=3/2
  Gain2 : Gain  Gain=1/2
  Product : Product  Inputs=3  Multiplication=Matrix(*)
  Subtract : Sum  Inputs=+-
  Transpose : Math  Operator=transpose
  Out1 : Outport
  wires:
  In1/1 -> Product/3, Product/1, Gain1/1, Transpose/1
  Gain2/1 -> Subtract/2
  Gain1/1 -> Subtract/1
  Product/1 -> Gain2/1
  Transpose/1 -> Product/2
  Subtract/1 -> Out1/1

== system Lab07/DCM/w^ ==
  In1 : Inport
  Constant3 : Constant  Value=0
  Constant4 : Constant  Value=0
  Constant5 : Constant  Value=0
  Demux : Demux  Outputs=3
  Gain : Gain  Gain=-1
  Gain1 : Gain  Gain=-1
  Gain2 : Gain  Gain=-1
  Matrix Concatenate : Concatenate  NumInputs=3  Mode=Multidimensional array  ConcatenateDimension=2
  Matrix Concatenate1 : Concatenate  NumInputs=3  Mode=Multidimensional array
  Matrix Concatenate2 : Concatenate  NumInputs=3  Mode=Multidimensional array
  Matrix Concatenate3 : Concatenate  NumInputs=3  Mode=Multidimensional array
  To Workspace : ToWorkspace  VariableName=merda  SampleTime=-1
  Out1 : Outport
  wires:
  Demux/3 -> Gain1/1, Matrix Concatenate1/2
  Constant4/1 -> Matrix Concatenate1/1
  Matrix Concatenate/1 -> To Workspace/1, Out1/1
  Demux/1 -> Gain2/1, Matrix Concatenate3/3
  Constant5/1 -> Matrix Concatenate3/2
  Matrix Concatenate1/1 -> Matrix Concatenate/1
  Constant3/1 -> Matrix Concatenate2/3
  Matrix Concatenate2/1 -> Matrix Concatenate/3
  Matrix Concatenate3/1 -> Matrix Concatenate/2
  Gain2/1 -> Matrix Concatenate2/2
  Demux/2 -> Matrix Concatenate2/1, Gain/1
  Gain1/1 -> Matrix Concatenate3/1
  Gain/1 -> Matrix Concatenate1/3
  In1/1 -> Demux/1

== system Lab07/SRP/Norm ==
  Vector : Inport
  Add : Sum  Inputs=+++
  Demux : Demux  Outputs=3
  Sqrt : Sqrt
  Square : Math  Operator=square
  Square1 : Math  Operator=square
  Square2 : Math  Operator=square
  Norm : Outport
  wires:
  Square/1 -> Add/1
  Add/1 -> Sqrt/1
  Demux/3 -> Square1/1
  Square2/1 -> Add/2
  Square1/1 -> Add/3
  Demux/1 -> Square/1
  Demux/2 -> Square2/1
  Vector/1 -> Demux/1
  Sqrt/1 -> Norm/1

== system Lab07/SRP/Norm1 ==
  Vector : Inport
  Add : Sum  Inputs=+++
  Demux : Demux  Outputs=3
  Sqrt : Sqrt
  Square : Math  Operator=square
  Square1 : Math  Operator=square
  Square2 : Math  Operator=square
  Norm : Outport
  wires:
  Square/1 -> Add/1
  Add/1 -> Sqrt/1
  Demux/3 -> Square1/1
  Square2/1 -> Add/2
  Square1/1 -> Add/3
  Demux/1 -> Square/1
  Demux/2 -> Square2/1
  Vector/1 -> Demux/1
  Sqrt/1 -> Norm/1

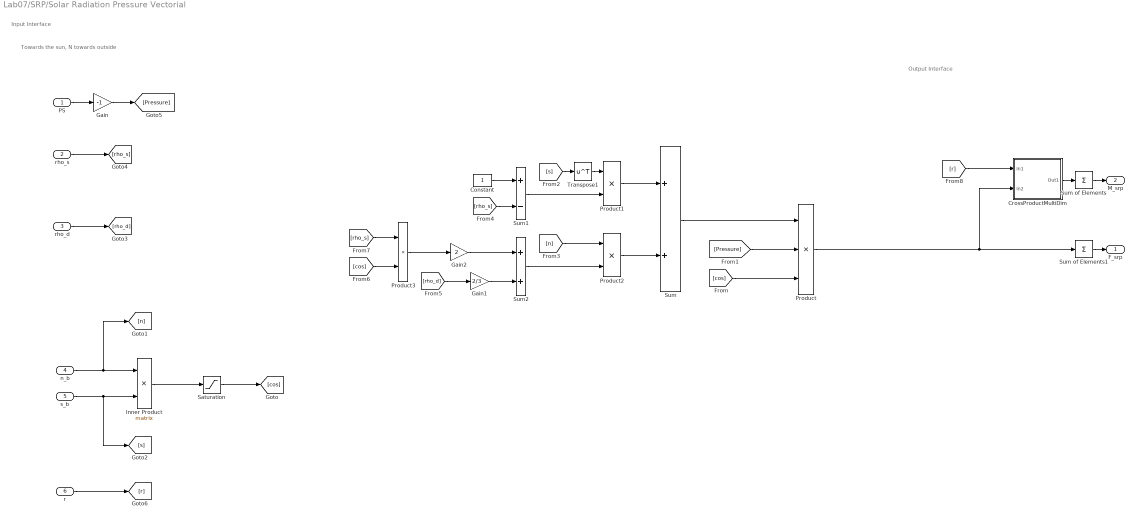
== system Lab07/SRP/Solar Radiation Pressure Vectorial ==
  note: Towards the sun, N towards outside
  note: Output Interface
  note: Input Interface
  PS : Inport
  rho_s : Inport  Port=2
  rho_d : Inport  Port=3
  n_b : Inport  Port=4
  s_b : Inport  Port=5
  r : Inport  Port=6
  Constant : Constant  VectorParams1D=off
  CrossProductMultiDim : Subsystem
  Gain : Gain  Gain=-1
  Gain1 : Gain  Gain=2/3
  Gain2 : Gain  Gain=2
  Inner Product : Product  Multiplication=Matrix(*)
  Product : Product  Inputs=3
  Product1 : Product
  Product2 : Product
  Product3 : Product
  Saturation : Saturate  UpperLimit=1  LowerLimit=0
  Sum : Sum
  Sum of Elements : Sum  Inputs=+
  Sum of Elements1 : Sum  Inputs=+
  Sum1 : Sum  Inputs=+-
  Sum2 : Sum
  Transpose1 : Math  Operator=transpose
  F_srp : Outport
  M_srp : Outport  Port=2
  wires:
  s_b/1 -> Inner Product/2, [s]
  n_b/1 -> Inner Product/1, [n]
  Saturation/1 -> [cos]
  PS/1 -> Gain/1
  Product/1 -> CrossProductMultiDim/2(In2), Sum of Elements1/1
  rho_d/1 -> [rho_d]
  rho_s/1 -> [rho_s]
  [cos] -> Product/3
  Gain/1 -> [Pressure]
  [Pressure] -> Product/2
  Sum/1 -> Product/1
  [s] -> Transpose1/1
  Product1/1 -> Sum/1
  Product2/1 -> Sum/2
  [n] -> Product2/1
  Sum1/1 -> Product1/2
  Sum2/1 -> Product2/2
  Constant/1 -> Sum1/1
  [rho_s] -> Sum1/2
  Gain1/1 -> Sum2/2
  [rho_d] -> Gain1/1
  Gain2/1 -> Sum2/1
  Product3/1 -> Gain2/1
  [cos] -> Product3/2
  [rho_s] -> Product3/1
  r/1 -> [r]
  [r] -> CrossProductMultiDim/1(In1)
  CrossProductMultiDim/1(Out1) -> Sum of Elements/1
  Sum of Elements/1 -> M_srp/1
  Sum of Elements1/1 -> F_srp/1
  Transpose1/1 -> Product1/1
  Inner Product/1 -> Saturation/1

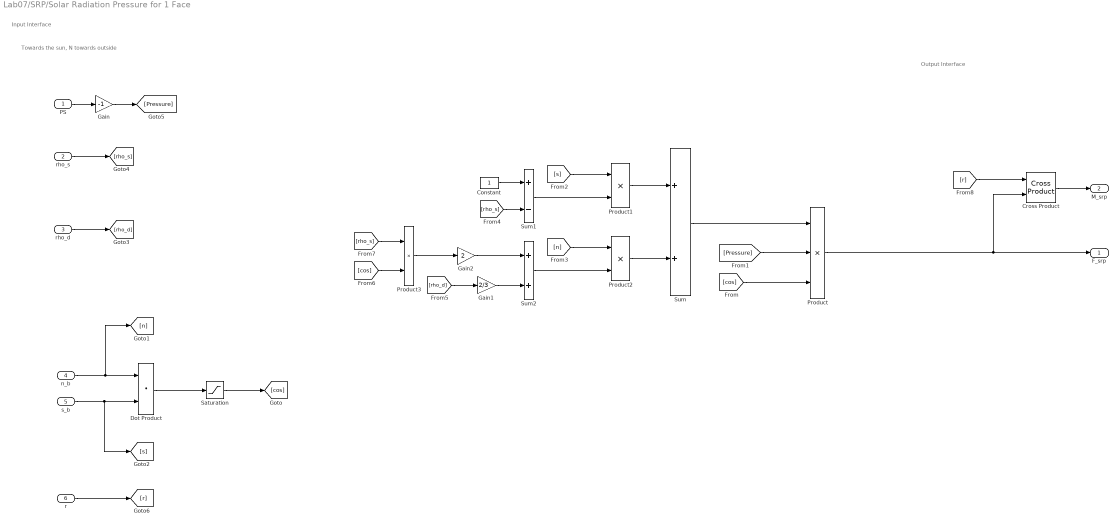
== system Lab07/SRP/Solar Radiation Pressure for 1 Face ==
  note: Towards the sun, N towards outside
  note: Output Interface
  note: Input Interface
  PS : Inport
  rho_s : Inport  Port=2
  rho_d : Inport  Port=3
  n_b : Inport  Port=4
  s_b : Inport  Port=5
  r : Inport  Port=6
  Constant : Constant
  Cross Product : matrix_library/Cross Product
  Dot Product : DotProduct  OutDataTypeStr=Inherit: Inherit via internal rule
  Gain : Gain  Gain=-1
  Gain1 : Gain  Gain=2/3
  Gain2 : Gain  Gain=2
  Product : Product  Inputs=3
  Product1 : Product
  Product2 : Product
  Product3 : Product
  Saturation : Saturate  UpperLimit=1  LowerLimit=0
  Sum : Sum
  Sum1 : Sum  Inputs=+-
  Sum2 : Sum
  F_srp : Outport
  M_srp : Outport  Port=2
  wires:
  s_b/1 -> [s], Dot Product/2
  n_b/1 -> [n], Dot Product/1
  Dot Product/1 -> Saturation/1
  Saturation/1 -> [cos]
  PS/1 -> Gain/1
  Product/1 -> Cross Product/2, F_srp/1
  rho_d/1 -> [rho_d]
  rho_s/1 -> [rho_s]
  [cos] -> Product/3
  Gain/1 -> [Pressure]
  [Pressure] -> Product/2
  Sum/1 -> Product/1
  [s] -> Product1/1
  Product1/1 -> Sum/1
  Product2/1 -> Sum/2
  [n] -> Product2/1
  Sum1/1 -> Product1/2
  Sum2/1 -> Product2/2
  Constant/1 -> Sum1/1
  [rho_s] -> Sum1/2
  Gain1/1 -> Sum2/2
  [rho_d] -> Gain1/1
  Gain2/1 -> Sum2/1
  Product3/1 -> Gain2/1
  [cos] -> Product3/2
  [rho_s] -> Product3/1
  r/1 -> [r]
  [r] -> Cross Product/1
  Cross Product/1 -> M_srp/1

== system Lab07/SRP/Solar Radiation Pressure Vectorial/CrossProductMultiDim ==
  In1 : Inport
  In2 : Inport  Port=2
  "A(:, t1)" : Selector  NumberOfDimensions=2  InputPortWidth=3  IndexOptions=Select all,Index vector (dialog)  Indices=[1 3],[2,3,1]  OutputSizes=1,1
  "A(:, t2)1" : Selector  NumberOfDimensions=2  InputPortWidth=3  IndexOptions=Select all,Index vector (dialog)  Indices=[1 3],[3,1,2]  OutputSizes=1,1
  "B(:, t1)" : Selector  NumberOfDimensions=2  InputPortWidth=3  IndexOptions=Select all,Index vector (dialog)  Indices=[1 3],[2,3,1]  OutputSizes=1,1
  "B(:, t2)" : Selector  NumberOfDimensions=2  InputPortWidth=3  IndexOptions=Select all,Index vector (dialog)  Indices=[1 3],[3,1,2]  OutputSizes=1,1
  Product : Product
  Product1 : Product
  Sum : Sum  Inputs=+-
  Out1 : Outport
  wires:
  In2/1 -> "B(:, t2)"/1, "B(:, t1)"/1
  In1/1 -> "A(:, t2)1"/1, "A(:, t1)"/1
  "A(:, t1)"/1 -> Product/2
  "B(:, t2)"/1 -> Product/1
  "A(:, t2)1"/1 -> Product1/1
  "B(:, t1)"/1 -> Product1/2
  Product/1 -> Sum/1
  Product1/1 -> Sum/2
  Sum/1 -> Out1/1
